simulink model "W02_S1"  (R2024b)
settings: Solver=ode4  StartTime=0  StopTime=T_final  FixedStep=h  RelTol=1e-3
values from neighbouring files (symbols this model uses):
  Kp = logspace(1.5, 4, 60)    [W02_S_expected.m]
undefined symbols (not defined in the file or in its folder): Kb, Kd, Ki, Nf, pid_b, pid_k, pid_m, t_step, tau_max, y_step
settings Model: Creator=admin  LastModifiedBy=admin
settings DataIOCC: ReturnWorkspaceOutputs=off

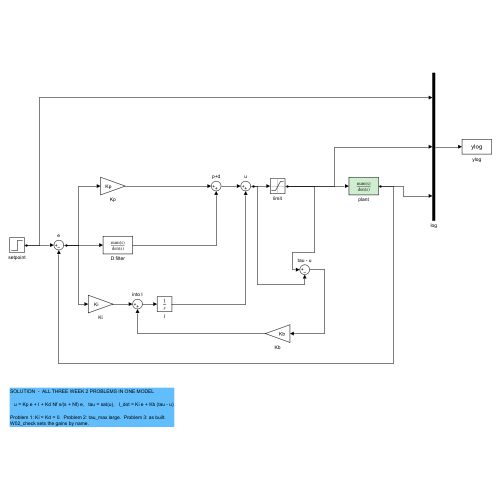
[thumbnail: Simulink's stored preview of the top-level diagram]
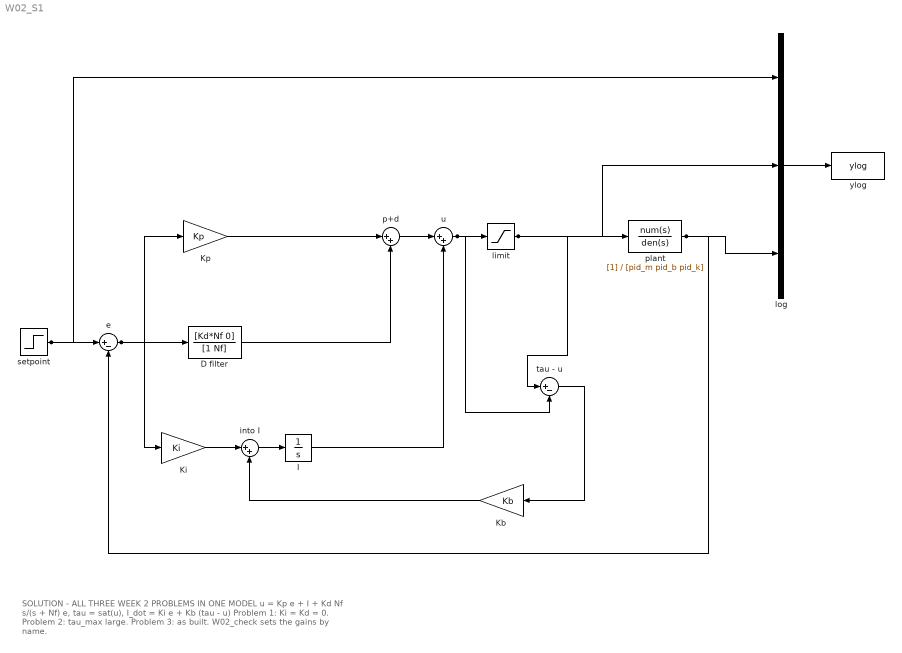
== system W02_S1 ==
  note: SOLUTION  -  ALL THREE WEEK 2 PROBLEMS IN ONE MODEL
      |
      |    u = Kp e + I + Kd Nf s/(s + Nf) e,   tau = sat(u),   I_dot = Ki e + Kb (tau - u)
      |
      | Problem 1: Ki = Kd = 0.  Problem 2: tau_max large.  Problem 3: as built.
      | W02_check sets the gains by name.
  D filter : TransferFcn  Numerator=[Kd*Nf 0]  Denominator=[1 Nf]
  I : Integrator
  Kb : Gain  Gain=Kb
  Ki : Gain  Gain=Ki
  Kp : Gain  Gain=Kp
  e : Sum  Inputs=|+-
  into I : Sum  Inputs=|++
  limit : Saturate  UpperLimit=tau_max  LowerLimit=-tau_max
  log : Mux  Inputs=3
  p+d : Sum  Inputs=|++
  plant : TransferFcn  Denominator=[pid_m pid_b pid_k]
  setpoint : Step  Time=t_step  After=y_step  SampleTime=0
  tau - u : Sum  Inputs=|+-
  u : Sum  Inputs=|++
  ylog : ToWorkspace  VariableName=ylog  SaveFormat=Structure With Time  SampleTime=-1
  wires:
  setpoint/1 -> e/1, log/1
  e/1 -> Kp/1, D filter/1, Ki/1
  Ki/1 -> into I/1
  into I/1 -> I/1
  Kp/1 -> p+d/1
  D filter/1 -> p+d/2
  p+d/1 -> u/1
  I/1 -> u/2
  u/1 -> limit/1, tau - u/2
  limit/1 -> plant/1, tau - u/1, log/2
  tau - u/1 -> Kb/1
  Kb/1 -> into I/2
  plant/1 -> e/2, log/3
  log/1 -> ylog/1
